simulink model "Drone_Control"  (R2022a)
settings: Solver=ode3  StartTime=0.0  StopTime=inf  RelTol=1e-3  EnableMultiTasking=on
settings Model: FPTRunName=Active  ExtModeTrigDuration=2  Creator=Rafael  LastModifiedBy=Rafael
settings SolverCC: AlgebraicLoopSolver=TrustRegion
settings DataIOCC: LimitDataPoints=on  SaveFormat=Array
settings OptimizationCC: ExpressionDepthLimit=2147483647  LifeSpan=Inf  MaxStackSize=64
settings DebuggingCC: UnderspecifiedInitializationDetection=Classic  MergeDetectMultiDrivingBlocksExec=none  FcnCallInpInsideContextMsg=warning  UnconnectedInputMsg=warning  UnconnectedOutputMsg=warning  UnconnectedLineMsg=warning  AllowSymbolicDim=off  StateNameClashWarn=warning  SFUnexpectedBacktrackingDiag=warning  SFNoUnconditionalDefaultTransitionDiag=warning  SFExecutionAtInitializationDiag=none  SFMachineParentedDataDiag=warning  ArithmeticOperatorsInVariantConditions=warning
settings HardwareCC: ProdBitPerPointer=32  ProdBitPerSizeT=32  ProdBitPerPtrDiffT=32  ProdLargestAtomicInteger=Long  ProdLargestAtomicFloat=Double  ProdWordSize=32  ProdHWDeviceType=ARM Compatible->ARM Cortex
settings ModelReferenceCC: PropagateSignalLabelsOutOfModel=off
settings SFSimCC: SimUseLocalCustomCode=off  CustomCodeUndefinedFunction=UseInterfaceOnly
settings RTWCC: SystemTargetFile=ert.tlc  HardwareBoard=Arduino Due  TemplateMakefile=ert_default_tmf  GenerateReport=on  RTWVerbose=off  RTWUseLocalCustomCode=off  Toolchain=Arduino ARM  BuildConfiguration=Faster Runs  LaunchReport=on  DLArmComputeVersion=19.05
settings CodeAppCC: ForceParamTrailComments=on  OperatorAnnotations=on  StateflowObjectComments=on  MATLABSourceComments=on
settings ERTTargetCC: MultiwordLength=2048  ERTCustomFileBanners=off  SupportContinuousTime=on  SupportNonInlinedSFcns=on  RemoveResetFunc=off  SupportVariableSizeSignals=on  ModelStepFunctionPrototypeControlCompliant=off  ExtModeTransport=3  ExtModeStaticAlloc=on  ExtModeStaticAllocSize=24576  ExtModeMexFile=ext_xcp  ExtModeIntrfLevel=Level2 - Open
settings ConfigComp: CovMetricSettings=dw  CovSaveCumulativeToWorkspaceVar=on  CovSaveSingleToWorkspaceVar=on  CovExternalEMLEnable=off  CovSFcnEnable=off

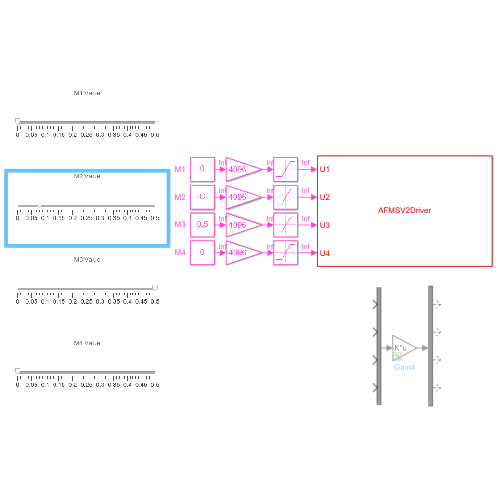
[thumbnail: Simulink's stored preview of the top-level diagram]
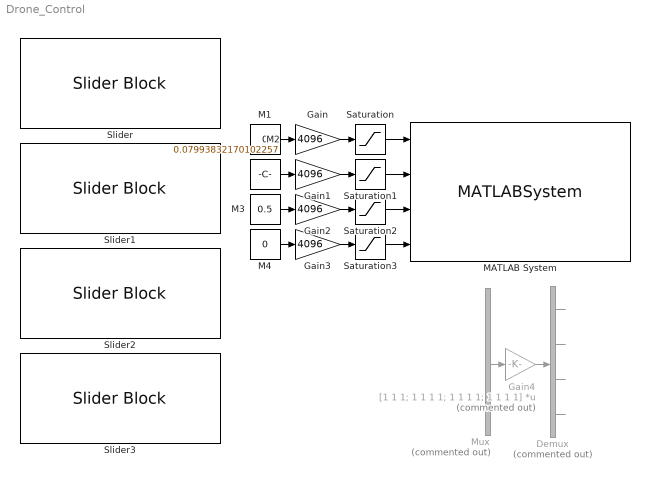
== system Drone_Control ==
  Demux : Demux  Commented=on
  Gain{,1..3} (4 alike) : Gain  Gain=4096
  Gain4 : Gain  Commented=on  Gain=[1 1 1; 1 1 1 1; 1 1 1 1; 1 1 1 1]  Multiplication=Matrix(K*u)
  M1 : Constant  Value=0
  M2 : Constant  Value=0.07993832170102257
  M3 : Constant  Value=0.5
  M4 : Constant  Value=0
  MATLAB System : MATLABSystem  System=AFMSV2Driver  SampleTime=0.1
      mask Type: AFMSV2Driver
      mask Display:
      | disp('AFMSV2Driver');
      | port_label('input',1,'U1');
      | port_label('input',2,'U2');
      | port_label('input',3,'U3');
      | port_label('input',4,'U4');
  Mux : Mux  Commented=on
  Saturation{,1..3} (4 alike) : Saturate  UpperLimit=1800  LowerLimit=0  OutDataTypeStr=int16
  Slider{,1..3} (4 alike) : SliderBlock  ScaleMax=0.5
  wires:
  Saturation/1 -> MATLAB System/1
  Saturation1/1 -> MATLAB System/2
  Saturation2/1 -> MATLAB System/3
  Saturation3/1 -> MATLAB System/4
  Gain/1 -> Saturation/1
  Gain1/1 -> Saturation1/1
  Gain2/1 -> Saturation2/1
  Gain3/1 -> Saturation3/1
  Mux/1 -> Gain4/1
  Demux/4 -> ?
  Demux/1 -> ?
  Demux/2 -> ?
  Gain4/1 -> Demux/1
  Demux/3 -> ?
  M1/1 -> Gain/1
  M2/1 -> Gain1/1
  M3/1 -> Gain2/1
  M4/1 -> Gain3/1
